simulink model "Lab4_LeadLag"  (R2016a)
settings: Solver=VariableStepAuto  StartTime=0.0  StopTime=60  RelTol=1e-3
libraries: simulink x2
settings Model: Creator=jordan  LastModifiedBy=jordan

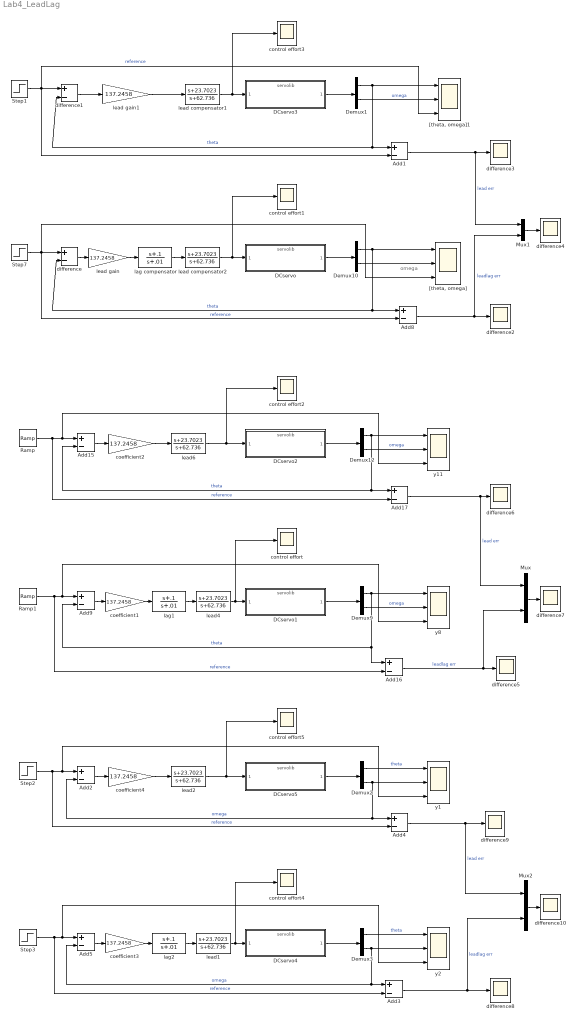
== system Lab4_LeadLag ==
  note: omega
  Add{1..5,8..9,15..17} (10 alike) : Sum  Inputs=+-
  DCservo{,1..5} (6 alike) : ModelReference  ModelNameDialog=servolib.slx  SimulationMode=Normal  ModelReferenceVersion=1.77
  Demux{1..3,9..10,12} (6 alike) : Demux  Outputs=2
  Mux : Mux  Inputs=2
  Mux1 : Mux  Inputs=2
  Mux2 : Mux  Inputs=2
  Ramp : simulink/Sources/Ramp  slope=1  start=0  X0=0
  Ramp1 : simulink/Sources/Ramp  slope=1  start=0  X0=0
  Step{1..3,7} (4 alike) : Step  SampleTime=0
  "[theta, omega]" : Scope  NumInputPorts=3
  "[theta, omega]1" : Scope  NumInputPorts=3
  coefficient{1..4} (4 alike) : Gain  Gain=137.2458
  control effort{,1..5} (6 alike) : Scope
  difference : Sum  Inputs=+-
  difference1 : Sum  Inputs=+-
  difference{2..10} (9 alike) : Scope
  lag compensator : TransferFcn  Numerator=[1 .1]  Denominator=[1 .01]
  lag1 : TransferFcn  Numerator=[1 .1]  Denominator=[1 .01]
  lag2 : TransferFcn  Numerator=[1 .1]  Denominator=[1 .01]
  lead compensator1 : TransferFcn  Numerator=[1 23.7023]  Denominator=[1 62.736]
  lead compensator2 : TransferFcn  Numerator=[1 23.7023]  Denominator=[1 62.736]
  lead gain : Gain  Gain=137.2458
  lead gain1 : Gain  Gain=137.2458
  lead{1..2,4,6} (4 alike) : TransferFcn  Numerator=[1 23.7023]  Denominator=[1 62.736]
  y{1..2,8,11} (4 alike) : Scope  NumInputPorts=3
  wires:
  lead compensator2/1 -> control effort1/1, DCservo/1
  Demux10/2 -> "[theta, omega]"/2
  difference/1 -> lead gain/1
  Step7/1 -> Add8/2, "[theta, omega]"/3, difference/1  "reference"
  Add8/1 -> difference2/1, Mux1/2  "leadlag err"
  Demux10/1 -> difference/2, Add8/1, "[theta, omega]"/1  "theta"
  lag compensator/1 -> lead compensator2/1
  lead gain/1 -> lag compensator/1
  DCservo/1 -> Demux10/1
  lead4/1 -> control effort/1, DCservo1/1
  Demux9/1 -> Add16/1, Add9/2, y8/1  "theta"
  Demux9/2 -> y8/2  "omega"
  Add9/1 -> coefficient1/1
  coefficient1/1 -> lag1/1
  lag1/1 -> lead4/1
  lead6/1 -> control effort2/1, DCservo2/1
  Demux12/1 -> Add17/1, Add15/2, y11/1  "theta"
  Demux12/2 -> y11/2  "omega"
  Add15/1 -> coefficient2/1
  coefficient2/1 -> lead6/1
  Ramp/1 -> Add17/2, y11/3, Add15/1  "reference"
  Add16/1 -> difference5/1, Mux/2  "leadlag err"
  Add17/1 -> Mux/1, difference6/1  "lead err"
  Mux/1 -> difference7/1
  Ramp1/1 -> Add16/2, y8/3, Add9/1  "reference"
  DCservo1/1 -> Demux9/1
  DCservo2/1 -> Demux12/1
  lead compensator1/1 -> control effort3/1, DCservo3/1
  Demux1/2 -> "[theta, omega]1"/2  "omega"
  difference1/1 -> lead gain1/1
  Step1/1 -> Add1/2, "[theta, omega]1"/3, difference1/1  "reference"
  Add1/1 -> Mux1/1, difference3/1  "lead err"
  Demux1/1 -> difference1/2, Add1/1, "[theta, omega]1"/1  "theta"
  lead gain1/1 -> lead compensator1/1
  DCservo3/1 -> Demux1/1
  Mux1/1 -> difference4/1
  lead1/1 -> control effort4/1, DCservo4/1
  Demux3/1 -> y2/1  "theta"
  Demux3/2 -> Add5/2, Add3/1, y2/2  "omega"
  Add5/1 -> coefficient3/1
  coefficient3/1 -> lag2/1
  lag2/1 -> lead1/1
  lead2/1 -> control effort5/1, DCservo5/1
  Demux2/1 -> y1/1  "theta"
  Demux2/2 -> Add2/2, Add4/1, y1/2  "omega"
  Add2/1 -> coefficient4/1
  coefficient4/1 -> lead2/1
  Step2/1 -> Add4/2, y1/3, Add2/1  "reference"
  Add3/1 -> difference8/1, Mux2/2  "leadlag err"
  Add4/1 -> difference9/1, Mux2/1  "lead err"
  Mux2/1 -> difference10/1
  Step3/1 -> Add3/2, y2/3, Add5/1  "reference"
  DCservo4/1 -> Demux3/1
  DCservo5/1 -> Demux2/1
